simulink model "Cold_Plate_test"  (R2014b)
settings: Solver=ode23tb  StartTime=0.0  StopTime=200  RelTol=1e-3
libraries: DAEMOT_Lib x3
settings Model: Creator=pangbor2  LastModifiedBy=pangbor2

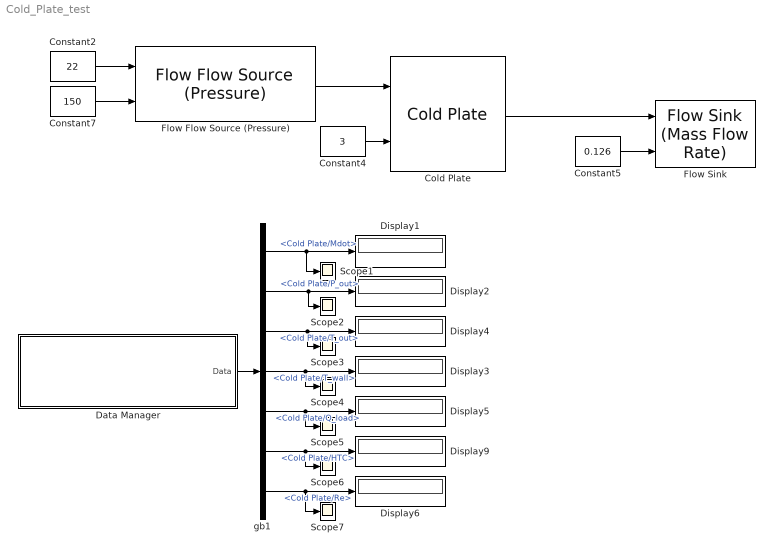
== system Cold_Plate_test ==
  Cold Plate : DAEMOT_Lib/Components/Cold Plate  fld=PG50  P_init=101  Tw_init=22  T_init=22  f=0.05  KL=0  PAF=1  M_wall=0.77632  Cp_wall=.9  D=0.007  L=0.75  t=0.0015  E=2.4e6  v=0.4  dH=-0.2  e_rough=0.0015*1e-3
  Constant2 : Constant  Value=22
  Constant4 : Constant  Value=3
  Constant5 : Constant  Value=0.126
  Constant7 : Constant  Value=150
  Data Manager : Subsystem  AncestorBlock=DAEMOT_Lib/Support Functions/Data Manager  mask{null=0}
      mask init:
      | set_param(gcb, 'LinkStatus', 'inactive')    % disable the library link
      settings: OpenFcn=data_manager
      mask Display: str ='Cold Plate/Mdot\nCold Plate/P_out\nCold Plate/T_out\nCold Plate/T_wall\nCold Plate/Q_load\nCold Plate/HTC\nCold Plate/Re'; fprintf(str)
  Display{1..6,9} (7 alike) : Display
  Flow Flow Source (Pressure) : DAEMOT_Lib/Components/Flow Flow Source (Pressure)  M_ext=on  M=0  T_ext=on  T=0  P_ext=on  P=0
  Flow Sink : DAEMOT_Lib/Components/Flow Sink (Mass Flow Rate)  M_ext=on  M=0  T_ext=on  T=0  P_ext=on  P=0
  Scope{1..7} (7 alike) : Scope
      Scope3 settings: SaveName=ScopeData2
      Scope4 settings: SaveName=ScopeData3
      Scope5 settings: SaveName=ScopeData4
      Scope6 settings: SaveName=ScopeData5
      Scope7 settings: SaveName=ScopeData6
  gb1 : BusSelector  OutputSignals=Cold Plate/Mdot,Cold Plate/P_out,Cold Plate/T_out,Cold Plate/T_wall,Cold Plate/Q_load,Cold Plate/HTC,Cold Plate/Re
  wires:
  Flow Flow Source (Pressure)/1 -> Cold Plate/1
  Constant5/1 -> Flow Sink/2
  Cold Plate/1 -> Flow Sink/1
  Constant4/1 -> Cold Plate/2
  Data Manager/1(Data) -> gb1/1
  gb1/1 -> Scope1/1, Display1/1  "<Cold Plate/Mdot>"
  gb1/2 -> Scope2/1, Display2/1  "<Cold Plate/P_out>"
  Constant7/1 -> Flow Flow Source (Pressure)/2
  Constant2/1 -> Flow Flow Source (Pressure)/1
  gb1/3 -> Scope3/1, Display4/1  "<Cold Plate/T_out>"
  gb1/4 -> Scope4/1, Display3/1  "<Cold Plate/T_wall>"
  gb1/5 -> Scope5/1, Display5/1  "<Cold Plate/Q_load>"
  gb1/6 -> Scope6/1, Display9/1  "<Cold Plate/HTC>"
  gb1/7 -> Scope7/1, Display6/1  "<Cold Plate/Re>"

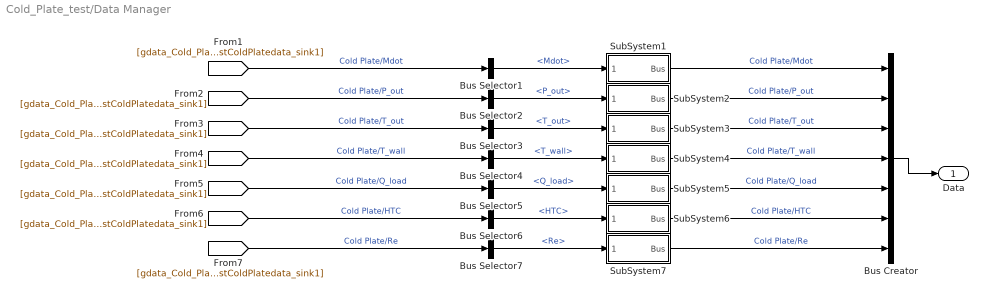
== system Cold_Plate_test/Data Manager ==
  Bus Creator : BusCreator  Inputs=7
  Bus Selector1 : BusSelector  OutputSignals=Mdot
  Bus Selector2 : BusSelector  OutputSignals=P_out
  Bus Selector3 : BusSelector  OutputSignals=T_out
  Bus Selector4 : BusSelector  OutputSignals=T_wall
  Bus Selector5 : BusSelector  OutputSignals=Q_load
  Bus Selector6 : BusSelector  OutputSignals=HTC
  Bus Selector7 : BusSelector  OutputSignals=Re
  SubSystem1 : Subsystem
  SubSystem2 : Subsystem
  SubSystem3 : Subsystem
  SubSystem4 : Subsystem
  SubSystem5 : Subsystem
  SubSystem6 : Subsystem
  SubSystem7 : Subsystem
  Data : Outport
  wires:
  Bus Creator/1 -> Data/1
  [gdata_Cold_Plate_testColdPlatedata_sink1] -> Bus Selector1/1  "Cold Plate/Mdot"
  Bus Selector1/1 -> SubSystem1/1(Rename)  "<Mdot>"
  SubSystem1/1(Bus) -> Bus Creator/1  "Cold Plate/Mdot"
  [gdata_Cold_Plate_testColdPlatedata_sink1] -> Bus Selector2/1  "Cold Plate/P_out"
  Bus Selector2/1 -> SubSystem2/1(Rename)  "<P_out>"
  SubSystem2/1(Bus) -> Bus Creator/2  "Cold Plate/P_out"
  [gdata_Cold_Plate_testColdPlatedata_sink1] -> Bus Selector3/1  "Cold Plate/T_out"
  Bus Selector3/1 -> SubSystem3/1(Rename)  "<T_out>"
  SubSystem3/1(Bus) -> Bus Creator/3  "Cold Plate/T_out"
  [gdata_Cold_Plate_testColdPlatedata_sink1] -> Bus Selector4/1  "Cold Plate/T_wall"
  Bus Selector4/1 -> SubSystem4/1(Rename)  "<T_wall>"
  SubSystem4/1(Bus) -> Bus Creator/4  "Cold Plate/T_wall"
  [gdata_Cold_Plate_testColdPlatedata_sink1] -> Bus Selector5/1  "Cold Plate/Q_load"
  Bus Selector5/1 -> SubSystem5/1(Rename)  "<Q_load>"
  SubSystem5/1(Bus) -> Bus Creator/5  "Cold Plate/Q_load"
  [gdata_Cold_Plate_testColdPlatedata_sink1] -> Bus Selector6/1  "Cold Plate/HTC"
  Bus Selector6/1 -> SubSystem6/1(Rename)  "<HTC>"
  SubSystem6/1(Bus) -> Bus Creator/6  "Cold Plate/HTC"
  [gdata_Cold_Plate_testColdPlatedata_sink1] -> Bus Selector7/1  "Cold Plate/Re"
  Bus Selector7/1 -> SubSystem7/1(Rename)  "<Re>"
  SubSystem7/1(Bus) -> Bus Creator/7  "Cold Plate/Re"

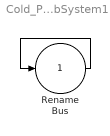
== system Cold_Plate_test/Data Manager/SubSystem1 ==
  Rename : Inport
  Bus : Outport
  wires:
  Rename/1 -> Bus/1

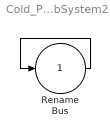
== system Cold_Plate_test/Data Manager/SubSystem2 ==
  Rename : Inport
  Bus : Outport
  wires:
  Rename/1 -> Bus/1

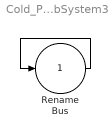
== system Cold_Plate_test/Data Manager/SubSystem3 ==
  Rename : Inport
  Bus : Outport
  wires:
  Rename/1 -> Bus/1

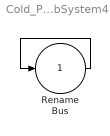
== system Cold_Plate_test/Data Manager/SubSystem4 ==
  Rename : Inport
  Bus : Outport
  wires:
  Rename/1 -> Bus/1

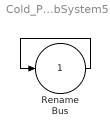
== system Cold_Plate_test/Data Manager/SubSystem5 ==
  Rename : Inport
  Bus : Outport
  wires:
  Rename/1 -> Bus/1

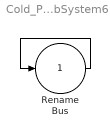
== system Cold_Plate_test/Data Manager/SubSystem6 ==
  Rename : Inport
  Bus : Outport
  wires:
  Rename/1 -> Bus/1

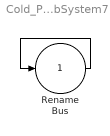
== system Cold_Plate_test/Data Manager/SubSystem7 ==
  Rename : Inport
  Bus : Outport
  wires:
  Rename/1 -> Bus/1
